simulink model "uas_sim"  (R2023a)
settings: Solver=VariableStepAuto  StartTime=0.0  StopTime=10.0  RelTol=1e-3  SampleTimeConstraint=STIndependent
values from neighbouring files (symbols this model uses):
  framePeriod_s = 1/frameRate_hz    (= 0.02)    [setup.m]
undefined symbols (not defined in the file or in its folder): Aircraft, datetime, datevec, Earth, Env, Fmu, InitCond, Telem, WGS84
libraries: aerolibconvert2 x8, simulink x8, aerolibadyn x3, aerolibasang x3, aerolibtransform2 x2, aerolibgravity2 x2, aerolibatmos2 x1, sharedutil x1, aerolibbdyn x1, shared6dof x1
(part 2 of 4)

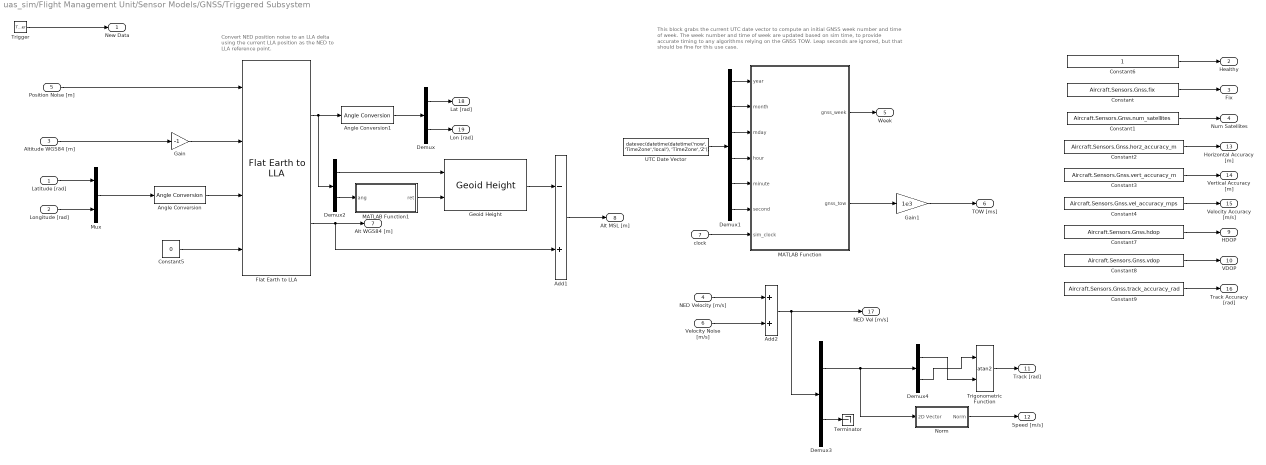
== system uas_sim/Flight Management Unit/Sensor Models/GNSS/Triggered Subsystem ==
  note: This block grabs the current UTC date vector to compute an initial GNSS week number
      | and time of week. The week number and time of week are updated based on sim time, to provide accurate timing to any algorithms relying on the GNSS TOW. Leap seconds are ignored, but that should be fine for this use case.
  note: Convert NED position noise to an LLA delta
      | using the current LLA position as the NED to
      | LLA reference point.
  Latitude [rad] : Inport
  "Longitude [rad] " : Inport  Port=2
  Altitude WGS84 [m] : Inport  Port=3
  NED Velocity [m/s] : Inport  Port=4  PortDimensions=3
  Position Noise [m] : Inport  Port=5  PortDimensions=3
  Velocity Noise [m/s] : Inport  Port=6  PortDimensions=3
  clock : Inport  Port=7
  Trigger : TriggerPort  VariantControl=Variant  ShowOutputPort=on
  Add1 : Sum  Inputs=-+
  Add2 : Sum
  Angle Conversion : aerolibconvert2/Angle Conversion  IU=rad  OU=deg
  Angle Conversion1 : aerolibconvert2/Angle Conversion  IU=deg  OU=rad
  Constant : Constant  Value=Aircraft.Sensors.Gnss.fix
  Constant1 : Constant  Value=Aircraft.Sensors.Gnss.num_satellites
  Constant2 : Constant  Value=Aircraft.Sensors.Gnss.horz_accuracy_m
  Constant3 : Constant  Value=Aircraft.Sensors.Gnss.vert_accuracy_m
  Constant4 : Constant  Value=Aircraft.Sensors.Gnss.vel_accuracy_mps
  Constant5 : Constant  Value=0
  Constant6 : Constant
  Constant7 : Constant  Value=Aircraft.Sensors.Gnss.hdop
  Constant8 : Constant  Value=Aircraft.Sensors.Gnss.vdop
  Constant9 : Constant  Value=Aircraft.Sensors.Gnss.track_accuracy_rad
  Demux : Demux  Outputs=2
  Demux1 : Demux  Outputs=6
  Demux2 : Demux  Outputs=2
  Demux3 : Demux  Outputs=[2 1]
  Demux4 : Demux  Outputs=2
  Flat Earth to LLA : aerolibtransform2/Flat Earth to LLA  units=Metric (MKS)  ptype=Earth (WGS84)  F=1/298.257223563  R=6378137  refPosPort=on  LL0=[0 10]  psi=0
  Gain : Gain  Gain=-1
  Gain1 : Gain  Gain=1e3
  Geoid Height : aerolibgravity2/Geoid Height  units=Metric (MKS)  gtype=EGM96  datafile='geoidegm96grid'  dtype=double  action=Warning
  MATLAB Function : MATLAB Function  TreatAsAtomicUnit=on
  MATLAB Function1 : MATLAB Function  TreatAsAtomicUnit=on
  Mux : Mux  Inputs=2
  Norm : Subsystem
  Terminator : Terminator
  Trigonometric Function : Trigonometry  Operator=atan2
  UTC Date Vector : Constant  Value=datevec(datetime(datetime('now', 'TimeZone','local'), 'TimeZone','Z'))  SampleTime=-1
  New Data : Outport
  Healthy : Outport  Port=2
  Fix : Outport  Port=3
  Num Satellites : Outport  Port=4
  Week : Outport  Port=5
  TOW [ms] : Outport  Port=6
  Alt WGS84 [m] : Outport  Port=7
  Alt MSL [m] : Outport  Port=8
  HDOP : Outport  Port=9
  VDOP : Outport  Port=10
  Track [rad] : Outport  Port=11
  Speed [m/s] : Outport  Port=12
  Horizontal Accuracy [m] : Outport  Port=13
  Vertical Accuracy [m] : Outport  Port=14
  Velocity Accuracy [m/s] : Outport  Port=15
  Track Accuracy [rad] : Outport  Port=16
  NED Vel [m/s] : Outport  Port=17
  Lat [rad] : Outport  Port=18
  Lon [rad] : Outport  Port=19
  wires:
  Constant/1 -> Fix/1
  Constant1/1 -> Num Satellites/1
  Constant2/1 -> Horizontal Accuracy [m]/1
  Constant3/1 -> Vertical Accuracy [m]/1
  Constant4/1 -> Velocity Accuracy [m/s]/1
  Position Noise [m]/1 -> Flat Earth to LLA/1
  Altitude WGS84 [m]/1 -> Gain/1
  Mux/1 -> Angle Conversion/1
  Angle Conversion/1 -> Flat Earth to LLA/3
  Constant5/1 -> Flat Earth to LLA/4
  "Longitude [rad] "/1 -> Mux/2
  Latitude [rad]/1 -> Mux/1
  Flat Earth to LLA/1 -> Demux2/1, Angle Conversion1/1
  Angle Conversion1/1 -> Demux/1
  Demux/2 -> Lon [rad]/1
  Demux/1 -> Lat [rad]/1
  Flat Earth to LLA/2 -> Add1/2, Alt WGS84 [m]/1
  NED Velocity [m/s]/1 -> Add2/1
  Add2/1 -> Demux3/1, NED Vel [m/s]/1
  Demux1/2 -> MATLAB Function/2(month)
  Demux1/6 -> MATLAB Function/6(second)
  UTC Date Vector/1 -> Demux1/1
  Demux1/1 -> MATLAB Function/1(year)
  Demux1/5 -> MATLAB Function/5(minute)
  Demux1/4 -> MATLAB Function/4(hour)
  Demux1/3 -> MATLAB Function/3(mday)
  MATLAB Function/2(gnss_tow) -> Gain1/1
  MATLAB Function/1(gnss_week) -> Week/1
  clock/1 -> MATLAB Function/7(sim_clock)
  Gain/1 -> Flat Earth to LLA/2
  Constant6/1 -> Healthy/1
  Trigger/1 -> New Data/1
  Gain1/1 -> TOW [ms]/1
  Demux2/1 -> Geoid Height/1
  Demux2/2 -> MATLAB Function1/1(ang)
  MATLAB Function1/1(ret) -> Geoid Height/2
  Geoid Height/1 -> Add1/1
  Add1/1 -> Alt MSL [m]/1
  Constant7/1 -> HDOP/1
  Constant8/1 -> VDOP/1
  Demux4/1 -> Trigonometric Function/2
  Demux4/2 -> Trigonometric Function/1
  Trigonometric Function/1 -> Track [rad]/1
  Velocity Noise [m/s]/1 -> Add2/2
  Constant9/1 -> Track Accuracy [rad]/1
  Demux3/1 -> Norm/1(2D Vector), Demux4/1
  Demux3/2 -> Terminator/1
  Norm/1(Norm) -> Speed [m/s]/1

== system uas_sim/Flight Management Unit/Sensor Models/IMU/Accelerometer ==
  Body Accel [m/s/s] : Inport  PortDimensions=3
  Gravitational Accel in Body Frame [m/s/s] : Inport  Port=2  PortDimensions=3
  Add : Sum  Inputs=+++
  Band-Limited White Noise : simulink/Sources/Band-Limited White Noise  Cov=Aircraft.Sensors.Imu.Accel.noise_mps2  Ts=0.1  seed=[23341]
  Constant : Constant  Value=Aircraft.Sensors.Imu.Accel.bias_mps2  VectorParams1D=off
  Constant1 : Constant  Value=Aircraft.Sensors.Imu.Accel.scale_factor
  Product : Product  Multiplication=Matrix(*)
  Reshape : Reshape  OutputDimensionality=Column vector (2-D)
  Reshape1 : Reshape  OutputDimensionality=Column vector (2-D)
  Reshape2 : Reshape
  Saturation : Saturate  UpperLimit=Aircraft.Sensors.Imu.Accel.upper_limit_mps2  LowerLimit=Aircraft.Sensors.Imu.Accel.lower_limit_mps2
  Subtract : Sum  Inputs=+-
  Accelerometer [m/s/s] : Outport  PortDimensions=3
  wires:
  Add/1 -> Saturation/1
  Band-Limited White Noise/1 -> Add/1
  Product/1 -> Add/3
  Constant/1 -> Add/2
  Constant1/1 -> Product/1
  Subtract/1 -> Product/2
  Reshape/1 -> Subtract/2
  Gravitational Accel in Body Frame [m/s/s]/1 -> Reshape/1
  Reshape1/1 -> Subtract/1
  Body Accel [m/s/s]/1 -> Reshape1/1
  Saturation/1 -> Reshape2/1
  Reshape2/1 -> Accelerometer [m/s/s]/1

== system uas_sim/Flight Management Unit/Sensor Models/IMU/Gyro ==
  Body Rotational Rate [rad/s] : Inport  PortDimensions=3
  Body Accel [m/s/s] : Inport  Port=2  PortDimensions=3
  Add1 : Sum  Inputs=++++
  Band-Limited White Noise : simulink/Sources/Band-Limited White Noise  Cov=Aircraft.Sensors.Imu.Gyro.noise_radps  Ts=0.1  seed=[23341]  VectorParams1D=off
  Constant1 : Constant  Value=Aircraft.Sensors.Imu.Gyro.bias_radps  VectorParams1D=off
  Constant2 : Constant  Value=Aircraft.Sensors.Imu.Gyro.accel_sens_radps
  Constant3 : Constant  Value=Aircraft.Sensors.Imu.Gyro.scale_factor  VectorParams1D=off
  Product : Product
  Product1 : Product  Multiplication=Matrix(*)
  Reshape : Reshape  OutputDimensionality=Column vector (2-D)
  Reshape1 : Reshape  OutputDimensionality=Column vector (2-D)
  Reshape2 : Reshape
  Saturation : Saturate  UpperLimit=Aircraft.Sensors.Imu.Gyro.upper_limit_radps  LowerLimit=Aircraft.Sensors.Imu.Gyro.lower_limit_radps
  Gyro [rad/s] : Outport  PortDimensions=3
  wires:
  Constant3/1 -> Product1/1
  Constant2/1 -> Product/1
  Add1/1 -> Saturation/1
  Constant1/1 -> Add1/3
  Product1/1 -> Add1/4
  Band-Limited White Noise/1 -> Add1/2
  Body Rotational Rate [rad/s]/1 -> Reshape/1
  Reshape/1 -> Product1/2
  Body Accel [m/s/s]/1 -> Product/2
  Product/1 -> Reshape1/1
  Reshape1/1 -> Add1/1
  Reshape2/1 -> Gyro [rad/s]/1
  Saturation/1 -> Reshape2/1

== system uas_sim/Flight Management Unit/Sensor Models/IMU/Magnetometer ==
  Body Magnetic Field [uT] : Inport  PortDimensions=3
  Add2 : Sum  Inputs=+++
  Band-Limited White Noise : simulink/Sources/Band-Limited White Noise  Cov=Aircraft.Sensors.Imu.Mag.noise_ut  Ts=0.1  seed=[23341]
  Constant1 : Constant  Value=Aircraft.Sensors.Imu.Mag.scale_factor  VectorParams1D=off
  Constant2 : Constant  Value=Aircraft.Sensors.Imu.Mag.bias_ut
  Product : Product  Multiplication=Matrix(*)
  Reshape : Reshape  OutputDimensionality=Column vector (2-D)
  Reshape1 : Reshape
  Saturation : Saturate  UpperLimit=Aircraft.Sensors.Imu.Mag.upper_limit_ut  LowerLimit=Aircraft.Sensors.Imu.Mag.lower_limit_ut
  Magnetometer [uT] : Outport  PortDimensions=3
  wires:
  Body Magnetic Field [uT]/1 -> Reshape/1
  Band-Limited White Noise/1 -> Add2/1
  Add2/1 -> Saturation/1
  Constant2/1 -> Add2/2
  Constant1/1 -> Product/1
  Reshape/1 -> Product/2
  Saturation/1 -> Reshape1/1
  Reshape1/1 -> Magnetometer [uT]/1
  Product/1 -> Add2/3

== system uas_sim/Flight Management Unit/Vehicle Management System (VMS)/Variant Subsystem/FMU v1 ==
  System Data : Inport
  Sensor Data : Inport  Port=2
  Navigation Filter Data : Inport  Port=3
  Telemetry Data : Inport  Port=4
  Flight Code : ModelReference  ModelNameDialog=fmu_v1.slx  SimulationMode=Normal  ModelReferenceVersion=2.2
  Virtual to Non-Virtual Mapping : Subsystem
  Virtual to Non-Virtual Mapping1 : Subsystem
  Virtual to Non-Virtual Mapping2 : Subsystem
  Virtual to Non-Virtual Mapping3 : Subsystem
  Virtual to Non-Virtual Mapping5 : Subsystem
  VMS Data : Outport
  wires:
  Telemetry Data/1 -> Virtual to Non-Virtual Mapping3/1(Virtual)
  Virtual to Non-Virtual Mapping2/1(Non-Virtual) -> Flight Code/3
  Virtual to Non-Virtual Mapping1/1(Non-Virtual) -> Flight Code/2
  Navigation Filter Data/1 -> Virtual to Non-Virtual Mapping2/1(Virtual)
  System Data/1 -> Virtual to Non-Virtual Mapping/1(Virtual)
  Flight Code/1 -> Virtual to Non-Virtual Mapping5/1(Non-Virtual)
  Virtual to Non-Virtual Mapping/1(Non-Virtual) -> Flight Code/1
  Virtual to Non-Virtual Mapping5/1(Virtual) -> VMS Data/1
  Sensor Data/1 -> Virtual to Non-Virtual Mapping1/1(Virtual)
  Virtual to Non-Virtual Mapping3/1(Non-Virtual) -> Flight Code/4

== system uas_sim/Flight Management Unit/Vehicle Management System (VMS)/Variant Subsystem/FMU v2 ==
  System Data : Inport
  Sensor Data : Inport  Port=2
  Navigation Filter Data : Inport  Port=3
  Telemetry Data : Inport  Port=4
  Flight Code : ModelReference  ModelNameDialog=fmu_v2.slx  SimulationMode=Normal  ModelReferenceVersion=4.2
  Virtual to Non-Virtual Mapping : Subsystem
  Virtual to Non-Virtual Mapping1 : Subsystem
  Virtual to Non-Virtual Mapping2 : Subsystem
  Virtual to Non-Virtual Mapping3 : Subsystem
  Virtual to Non-Virtual Mapping4 : Subsystem
  VMS Data : Outport
  wires:
  Virtual to Non-Virtual Mapping3/1(Non-Virtual) -> Flight Code/4
  Sensor Data/1 -> Virtual to Non-Virtual Mapping1/1(Virtual)
  Virtual to Non-Virtual Mapping4/1(Virtual) -> VMS Data/1
  Virtual to Non-Virtual Mapping/1(Non-Virtual) -> Flight Code/1
  Flight Code/1 -> Virtual to Non-Virtual Mapping4/1(Non-Virtual)
  System Data/1 -> Virtual to Non-Virtual Mapping/1(Virtual)
  Navigation Filter Data/1 -> Virtual to Non-Virtual Mapping2/1(Virtual)
  Virtual to Non-Virtual Mapping1/1(Non-Virtual) -> Flight Code/2
  Virtual to Non-Virtual Mapping2/1(Non-Virtual) -> Flight Code/3
  Telemetry Data/1 -> Virtual to Non-Virtual Mapping3/1(Virtual)

== system uas_sim/Flight Management Unit/Vehicle Management System (VMS)/Variant Subsystem/FMU v2 Beta ==
  System Data : Inport
  Sensor Data : Inport  Port=2
  Navigation Filter Data : Inport  Port=3
  Telemetry Data : Inport  Port=4
  Flight Code : ModelReference  ModelNameDialog=fmu_v2_beta.slx  SimulationMode=Normal  ModelReferenceVersion=2.5
  Virtual to Non-Virtual Mapping : Subsystem
  Virtual to Non-Virtual Mapping1 : Subsystem
  Virtual to Non-Virtual Mapping2 : Subsystem
  Virtual to Non-Virtual Mapping3 : Subsystem
  Virtual to Non-Virtual Mapping5 : Subsystem
  VMS Data : Outport
  wires:
  Virtual to Non-Virtual Mapping3/1(Non-Virtual) -> Flight Code/4
  Sensor Data/1 -> Virtual to Non-Virtual Mapping1/1(Virtual)
  Virtual to Non-Virtual Mapping5/1(Virtual) -> VMS Data/1
  Virtual to Non-Virtual Mapping/1(Non-Virtual) -> Flight Code/1
  Flight Code/1 -> Virtual to Non-Virtual Mapping5/1(Non-Virtual)
  System Data/1 -> Virtual to Non-Virtual Mapping/1(Virtual)
  Navigation Filter Data/1 -> Virtual to Non-Virtual Mapping2/1(Virtual)
  Virtual to Non-Virtual Mapping1/1(Non-Virtual) -> Flight Code/2
  Virtual to Non-Virtual Mapping2/1(Non-Virtual) -> Flight Code/3
  Telemetry Data/1 -> Virtual to Non-Virtual Mapping3/1(Virtual)

== system uas_sim/Vehicle/Forces and Moments/Aerodynamic/Aerodynamic Forces and Moments Coef Axis Variant ==
  Coef : Inport
  Dynamic Pressure [Pa] : Inport  Port=2
  Body Velocity [m/s] : Inport  Port=3
  Body Axis Coef : Subsystem  VariantControl=Aircraft.Aero.axis == 3
  Stability Axis Coef : Subsystem  VariantControl=Aircraft.Aero.axis == 2
  Wind Axis Coef : Subsystem  VariantControl=Aircraft.Aero.axis == 1
  Fxyz Mxyz : Outport

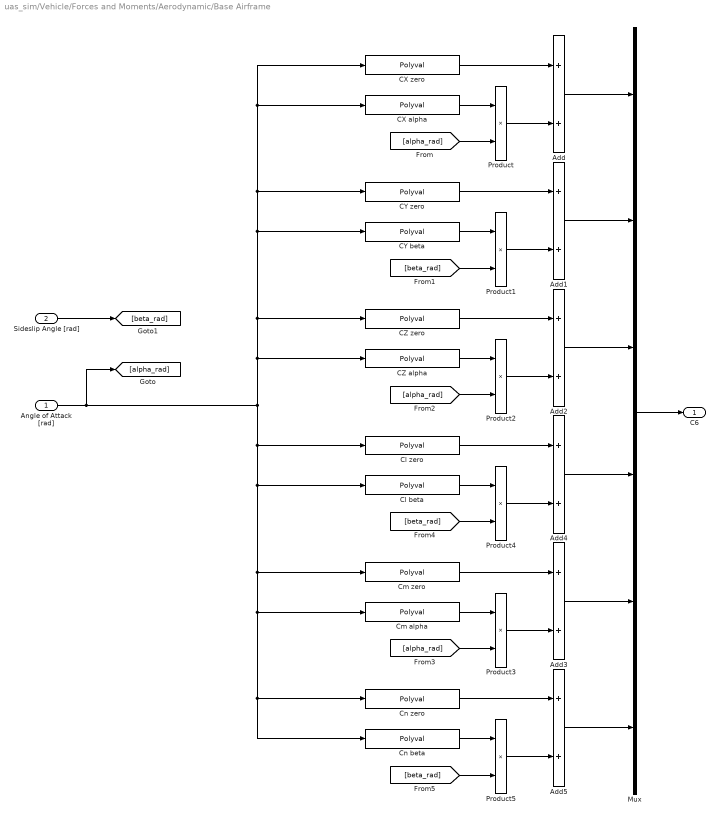
== system uas_sim/Vehicle/Forces and Moments/Aerodynamic/Base Airframe ==
  Angle of Attack [rad] : Inport
  Sideslip Angle [rad] : Inport  Port=2
  Add{,1..5} (6 alike) : Sum
  CX alpha : Polyval  Coefs=Aircraft.Aero.CX.alpha
  CX zero : Polyval  Coefs=Aircraft.Aero.CX.zero
  CY beta : Polyval  Coefs=Aircraft.Aero.CY.beta
  CY zero : Polyval  Coefs=Aircraft.Aero.CY.zero
  CZ alpha : Polyval  Coefs=Aircraft.Aero.CZ.alpha
  CZ zero : Polyval  Coefs=Aircraft.Aero.CZ.zero
  Cl beta : Polyval  Coefs=Aircraft.Aero.Cl.beta
  Cl zero : Polyval  Coefs=Aircraft.Aero.Cl.zero
  Cm alpha : Polyval  Coefs=Aircraft.Aero.Cm.alpha
  Cm zero : Polyval  Coefs=Aircraft.Aero.Cm.zero
  Cn beta : Polyval  Coefs=Aircraft.Aero.Cn.beta
  Cn zero : Polyval  Coefs=Aircraft.Aero.Cn.zero
  Mux : Mux  Inputs=6
  Product{,1..5} (6 alike) : Product
  C6 : Outport
  wires:
  Product/1 -> Add/2
  Add/1 -> Mux/1
  CX alpha/1 -> Product/1
  CX zero/1 -> Add/1
  Sideslip Angle [rad]/1 -> [beta_rad]
  [alpha_rad] -> Product/2
  Mux/1 -> C6/1
  [beta_rad] -> Product1/2
  CY zero/1 -> Add1/1
  CY beta/1 -> Product1/1
  Product1/1 -> Add1/2
  Add1/1 -> Mux/2
  CZ zero/1 -> Add2/1
  CZ alpha/1 -> Product2/1
  Add2/1 -> Mux/3
  Product2/1 -> Add2/2
  Product3/1 -> Add3/2
  Add3/1 -> Mux/5
  Cm alpha/1 -> Product3/1
  Cm zero/1 -> Add3/1
  [alpha_rad] -> Product2/2
  [alpha_rad] -> Product3/2
  Add4/1 -> Mux/4
  Product4/1 -> Add4/2
  Cl beta/1 -> Product4/1
  Cl zero/1 -> Add4/1
  [beta_rad] -> Product4/2
  [beta_rad] -> Product5/2
  Cn zero/1 -> Add5/1
  Cn beta/1 -> Product5/1
  Product5/1 -> Add5/2
  Add5/1 -> Mux/6
  Angle of Attack [rad]/1 -> [alpha_rad], Cl zero/1, Cl beta/1, Cm zero/1, Cm alpha/1, Cn zero/1, Cn beta/1, CZ alpha/1, CZ zero/1, CY beta/1, CY zero/1, CX alpha/1, CX zero/1

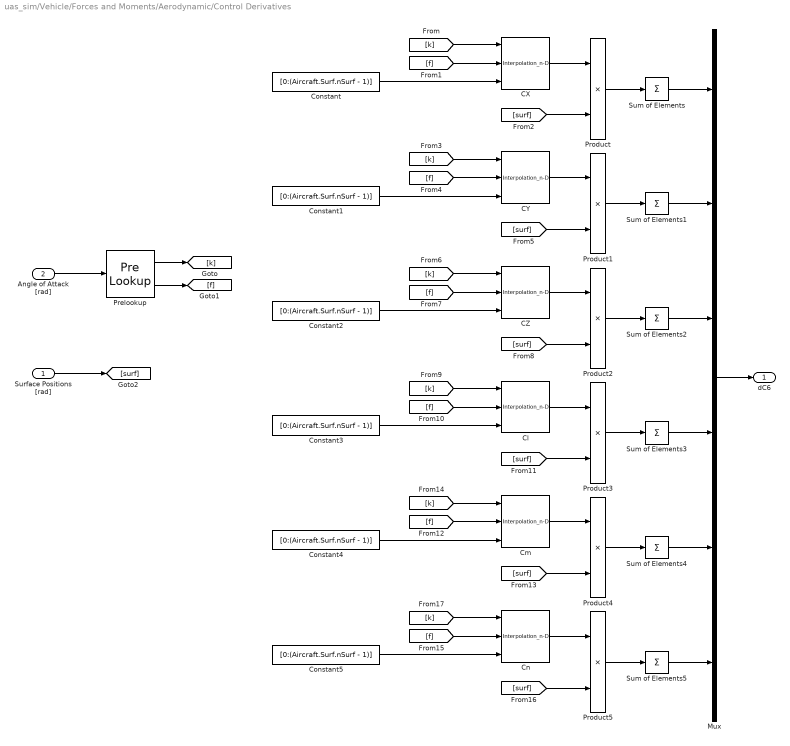
== system uas_sim/Vehicle/Forces and Moments/Aerodynamic/Control Derivatives ==
  Surface Positions [rad] : Inport
  Angle of Attack [rad] : Inport  Port=2
  CX : Interpolation_n-D  Table=Aircraft.Aero.CX.surf  DiagnosticForOutOfRangeInput=Warning  NumSelectionDims=1  InternalRulePriority=Speed
      settings: InputPortMap=u0,u1,u2
  CY : Interpolation_n-D  Table=Aircraft.Aero.CY.surf  DiagnosticForOutOfRangeInput=Warning  NumSelectionDims=1  InternalRulePriority=Speed
      settings: InputPortMap=u0,u1,u2
  CZ : Interpolation_n-D  Table=Aircraft.Aero.CZ.surf  DiagnosticForOutOfRangeInput=Warning  NumSelectionDims=1  InternalRulePriority=Speed
      settings: InputPortMap=u0,u1,u2
  Cl : Interpolation_n-D  Table=Aircraft.Aero.Cl.surf  DiagnosticForOutOfRangeInput=Warning  NumSelectionDims=1  InternalRulePriority=Speed
      settings: InputPortMap=u0,u1,u2
  Cm : Interpolation_n-D  Table=Aircraft.Aero.Cm.surf  DiagnosticForOutOfRangeInput=Warning  NumSelectionDims=1  InternalRulePriority=Speed
      settings: InputPortMap=u0,u1,u2
  Cn : Interpolation_n-D  Table=Aircraft.Aero.Cn.surf  DiagnosticForOutOfRangeInput=Warning  NumSelectionDims=1  InternalRulePriority=Speed
      settings: InputPortMap=u0,u1,u2
  Constant{,1..5} (6 alike) : Constant  Value=[0:(Aircraft.Surf.nSurf - 1)]
  Mux : Mux  Inputs=6
  Prelookup : PreLookup  BreakpointsData=Aircraft.Aero.CntrlEff.alpha  ExtrapMethod=Linear
  Product{,1..5} (6 alike) : Product
  Sum of Elements{,1..5} (6 alike) : Sum  Inputs=+
  dC6 : Outport
  wires:
  [k] -> Cm/1
  CY/1 -> Product1/1
  [f] -> Cn/2
  Product5/1 -> Sum of Elements5/1
  [surf] -> Product5/2
  Constant4/1 -> Cm/3
  Sum of Elements1/1 -> Mux/2
  [k] -> Cn/1
  Sum of Elements5/1 -> Mux/6
  Constant3/1 -> Cl/3
  [surf] -> Product3/2
  [k] -> Cl/1
  [f] -> Cl/2
  Constant2/1 -> CZ/3
  [k] -> CZ/1
  [surf] -> Product2/2
  Cl/1 -> Product3/1
  CZ/1 -> Product2/1
  Product2/1 -> Sum of Elements2/1
  Product3/1 -> Sum of Elements3/1
  Product1/1 -> Sum of Elements1/1
  Product/1 -> Sum of Elements/1
  [k] -> CY/1
  [f] -> CY/2
  Constant1/1 -> CY/3
  Constant/1 -> CX/3
  Cm/1 -> Product4/1
  [k] -> CX/1
  [surf] -> Product/2
  Prelookup/2 -> [f]
  Mux/1 -> dC6/1
  Prelookup/1 -> [k]
  Product4/1 -> Sum of Elements4/1
  Cn/1 -> Product5/1
  Angle of Attack [rad]/1 -> Prelookup/1
  Surface Positions [rad]/1 -> [surf]
  [f] -> CZ/2
  [f] -> Cm/2
  Sum of Elements2/1 -> Mux/3
  CX/1 -> Product/1
  [f] -> CX/2
  Constant5/1 -> Cn/3
  [surf] -> Product4/2
  Sum of Elements/1 -> Mux/1
  Sum of Elements4/1 -> Mux/5
  [surf] -> Product1/2
  Sum of Elements3/1 -> Mux/4

== system uas_sim/Vehicle/Forces and Moments/Aerodynamic/Dynamic Derivatives ==
  note: Divide by zero protection
  Airspeed [m/s] : Inport
  Body Rotational Rate [rad/s] : Inport  Port=2
  Angle of Attack [rad] : Inport  Port=3
  Add : Sum  Inputs=+++
  Constant : Constant  Value=Aircraft.Geom.b_m
  Constant1 : Constant  Value=Aircraft.Geom.c_m
  Constant2 : Constant  Value=Aircraft.Geom.b_m
  Demux : Demux  Outputs=3
  Divide : Product  Inputs=*/
  Gain : Gain  Gain=2
  Mux : Mux  Inputs=3
  Pitch Rate : Subsystem
  Product : Product
  Roll Rate : Subsystem
  Saturation : Saturate  UpperLimit=inf  LowerLimit=1e-3
  Yaw Rate : Subsystem
  dC6 : Outport
  wires:
  Constant/1 -> Mux/1
  Body Rotational Rate [rad/s]/1 -> Product/1
  Mux/1 -> Product/2
  Airspeed [m/s]/1 -> Gain/1
  Gain/1 -> Saturation/1
  Product/1 -> Divide/1
  Saturation/1 -> Divide/2
  Divide/1 -> Demux/1
  Demux/1 -> Roll Rate/2(p_hat)
  Demux/2 -> Pitch Rate/2(q_hat)
  Demux/3 -> Yaw Rate/2(r_hat)
  Angle of Attack [rad]/1 -> Yaw Rate/1(Angle of Attack [rad]), Pitch Rate/1(Angle of Attack [rad]), Roll Rate/1(Angle of Attack [rad])
  Roll Rate/1(dC6) -> Add/1
  Pitch Rate/1(dC6) -> Add/2
  Yaw Rate/1(dC6) -> Add/3
  Constant2/1 -> Mux/3
  Constant1/1 -> Mux/2
  Add/1 -> dC6/1

== system uas_sim/Vehicle/Forces and Moments/Propulsive/Motor ==
  note: RPM to rad/s
  Voltage [V] : Inport
  Motor Rotation Rate [rad/s] : Inport  Port=2
  Constant : Constant  Value=Aircraft.Motor.kv
  Constant1 : Constant  Value=Aircraft.Motor.io
  Divide : Product  Inputs=*/
  Divide2 : Product  Inputs=*/
  Gain : Gain  Gain=1/Aircraft.Motor.r
  Gain2 : Gain  Gain=2 * pi / 60
  Subtract : Sum  Inputs=+-
  Subtract1 : Sum  Inputs=+-
  Torque [N-m] : Outport
  wires:
  Gain2/1 -> [KvSI], Divide/2
  [KvSI] -> Divide2/2
  Constant1/1 -> Subtract1/2
  Motor Rotation Rate [rad/s]/1 -> Divide/1
  Divide/1 -> Subtract/2
  Constant/1 -> Gain2/1
  Gain/1 -> Subtract1/1
  Subtract1/1 -> Divide2/1
  Voltage [V]/1 -> Subtract/1
  Divide2/1 -> Torque [N-m]/1
  Subtract/1 -> Gain/1

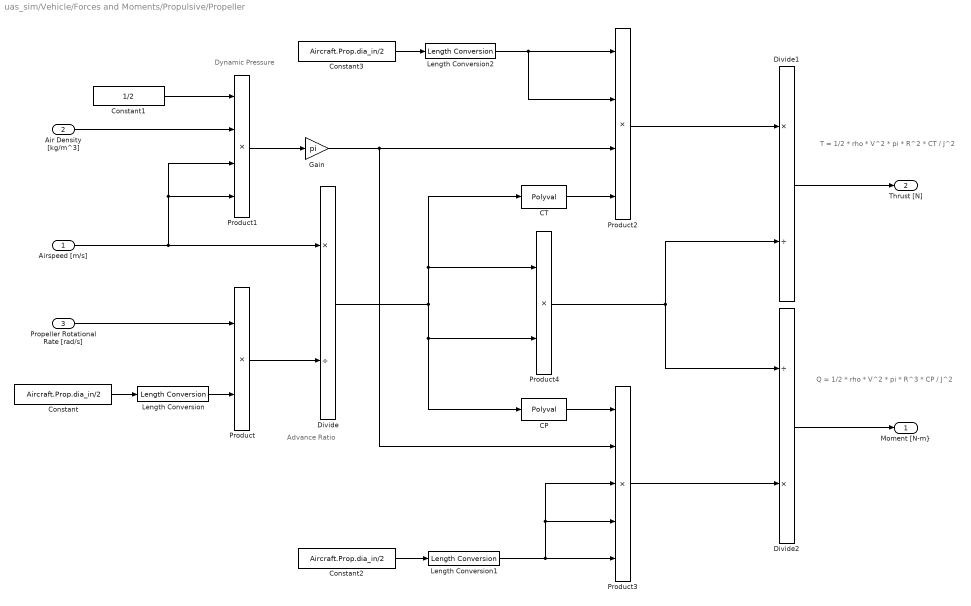
== system uas_sim/Vehicle/Forces and Moments/Propulsive/Propeller ==
  note: Dynamic Pressure
  note: Q = 1/2 * rho * V^2 * pi * R^3 * CP / J^2
  note: T = 1/2 * rho * V^2 * pi * R^2 * CT / J^2
  note: Advance Ratio
  Airspeed [m/s] : Inport
  Air Density [kg/m^3] : Inport  Port=2
  Propeller Rotational Rate [rad/s] : Inport  Port=3
  CP : Polyval  Coefs=Aircraft.prop.cp
  CT : Polyval  Coefs=Aircraft.prop.ct
  Constant : Constant  Value=Aircraft.Prop.dia_in/2
  Constant1 : Constant  Value=1/2
  Constant2 : Constant  Value=Aircraft.Prop.dia_in/2
  Constant3 : Constant  Value=Aircraft.Prop.dia_in/2
  Divide : Product  Inputs=*/
  Divide1 : Product  Inputs=*/
  Divide2 : Product  Inputs=/*
  Gain : Gain  Gain=pi
  Length Conversion : aerolibconvert2/Length Conversion  IU=in  OU=m
  Length Conversion1 : aerolibconvert2/Length Conversion  IU=in  OU=m
  Length Conversion2 : aerolibconvert2/Length Conversion  IU=in  OU=m
  Product : Product
  Product1 : Product  Inputs=4
  Product2 : Product  Inputs=4
  Product3 : Product  Inputs=5
  Product4 : Product
  "Moment [N-m}" : Outport
  Thrust [N] : Outport  Port=2
  wires:
  Divide2/1 -> "Moment [N-m}"/1
  Length Conversion/1 -> Product/2
  Product4/1 -> Divide2/1, Divide1/2
  Constant2/1 -> Length Conversion1/1
  Airspeed [m/s]/1 -> Divide/1, Product1/4, Product1/3
  Propeller Rotational Rate [rad/s]/1 -> Product/1
  Length Conversion1/1 -> Product3/4, Product3/3, Product3/5
  Product1/1 -> Gain/1
  Gain/1 -> Product3/2, Product2/3
  Air Density [kg/m^3]/1 -> Product1/2
  Divide1/1 -> Thrust [N]/1
  Product3/1 -> Divide2/2
  Constant1/1 -> Product1/1
  CP/1 -> Product3/1
  CT/1 -> Product2/4
  Product2/1 -> Divide1/1
  Length Conversion2/1 -> Product2/2, Product2/1
  Constant/1 -> Length Conversion/1
  Constant3/1 -> Length Conversion2/1
  Divide/1 -> Product4/2, CP/1, Product4/1, CT/1
  Product/1 -> Divide/2

== system uas_sim/Flight Management Unit/Sensor Models/GNSS/Triggered Subsystem/Norm ==
  2D Vector : Inport
  Product : Product
  Sqrt : Sqrt
  Sum of Elements : Sum  Inputs=+
  Norm : Outport
  wires:
  2D Vector/1 -> Product/2, Product/1
  Product/1 -> Sum of Elements/1
  Sum of Elements/1 -> Sqrt/1
  Sqrt/1 -> Norm/1

== system uas_sim/Flight Management Unit/Vehicle Management System (VMS)/Variant Subsystem/FMU v1/Virtual to Non-Virtual Mapping ==
  Virtual : Inport
  Bus Creator : BusCreator  Inputs=6  OutDataTypeStr=Bus: SysData  NonVirtualBus=on
  Bus Selector : BusSelector  OutputSignals=Frame Time [us],Input Voltage,Regulated Voltage,PWM Voltage,SBUS Voltage,System Time [us]
  Data Type Conversion : DataTypeConversion  OutDataTypeStr=int32  SaturateOnIntegerOverflow=off  RndMeth=Floor
  Data Type Conversion{1..4} (4 alike) : DataTypeConversion  OutDataTypeStr=single  SaturateOnIntegerOverflow=off  RndMeth=Floor
  Data Type Conversion5 : DataTypeConversion  OutDataTypeStr=int64  SaturateOnIntegerOverflow=off  RndMeth=Floor
  Non-Virtual : Outport  OutDataTypeStr=Bus: SysData
  wires:
  Data Type Conversion5/1 -> Bus Creator/6  "sys_time_us"
  Bus Selector/6 -> Data Type Conversion5/1  "<System Time [us]>"
  Data Type Conversion4/1 -> Bus Creator/5  "sbus_volt"
  Data Type Conversion3/1 -> Bus Creator/4  "pwm_volt"
  Data Type Conversion2/1 -> Bus Creator/3  "reg_volt"
  Bus Selector/5 -> Data Type Conversion4/1  "<SBUS Voltage>"
  Bus Selector/4 -> Data Type Conversion3/1  "<PWM Voltage>"
  Bus Selector/3 -> Data Type Conversion2/1  "<Regulated Voltage>"
  Data Type Conversion1/1 -> Bus Creator/2  "input_volt"
  Bus Selector/2 -> Data Type Conversion1/1  "<Input Voltage>"
  Data Type Conversion/1 -> Bus Creator/1  "frame_time_us"
  Bus Selector/1 -> Data Type Conversion/1  "<Frame Time [us]>"
  Virtual/1 -> Bus Selector/1
  Bus Creator/1 -> Non-Virtual/1

== system uas_sim/Flight Management Unit/Vehicle Management System (VMS)/Variant Subsystem/FMU v1/Virtual to Non-Virtual Mapping1 ==
  Virtual : Inport
  Bus Creator : BusCreator  Inputs=7  OutDataTypeStr=Bus: SensorData  NonVirtualBus=on
  Bus Selector : BusSelector  OutputSignals=Pitot Static Installed,Inceptor,IMU,GNSS,Static Pressure,Differential Pressure,Analog
  Data Type Conversion : DataTypeConversion  OutDataTypeStr=boolean  SaturateOnIntegerOverflow=off  RndMeth=Floor
  Virtual to Non-Virtual Mapping1 : Subsystem
  Virtual to Non-Virtual Mapping2 : Subsystem
  Virtual to Non-Virtual Mapping3 : Subsystem
  Virtual to Non-Virtual Mapping4 : Subsystem
  Virtual to Non-Virtual Mapping5 : Subsystem
  Virtual to Non-Virtual Mapping6 : Subsystem
  Non-Virtual : Outport  OutDataTypeStr=Bus: SensorData
  wires:
  Virtual/1 -> Bus Selector/1
  Bus Creator/1 -> Non-Virtual/1
  Bus Selector/1 -> Data Type Conversion/1  "<Pitot Static Installed>"
  Data Type Conversion/1 -> Bus Creator/1  "pitot_static_installed"
  Bus Selector/2 -> Virtual to Non-Virtual Mapping1/1(Virtual)  "<Inceptor>"
  Virtual to Non-Virtual Mapping1/1(Non-Virtual) -> Bus Creator/2  "inceptor"
  Virtual to Non-Virtual Mapping2/1(Non-Virtual) -> Bus Creator/3  "imu"
  Bus Selector/3 -> Virtual to Non-Virtual Mapping2/1(Virtual)  "<IMU>"
  Virtual to Non-Virtual Mapping3/1(Non-Virtual) -> Bus Creator/4  "gnss"
  Bus Selector/4 -> Virtual to Non-Virtual Mapping3/1(Virtual)  "<GNSS>"
  Virtual to Non-Virtual Mapping4/1(Non-Virtual) -> Bus Creator/5  "static_pres"
  Bus Selector/5 -> Virtual to Non-Virtual Mapping4/1(Virtual)  "<Static Pressure>"
  Virtual to Non-Virtual Mapping5/1(Non-Virtual) -> Bus Creator/6  "diff_pres"
  Bus Selector/6 -> Virtual to Non-Virtual Mapping5/1(Virtual)  "<Differential Pressure>"
  Bus Selector/7 -> Virtual to Non-Virtual Mapping6/1(Virtual)  "<Analog>"
  Virtual to Non-Virtual Mapping6/1(Non-Virtual) -> Bus Creator/7  "adc"

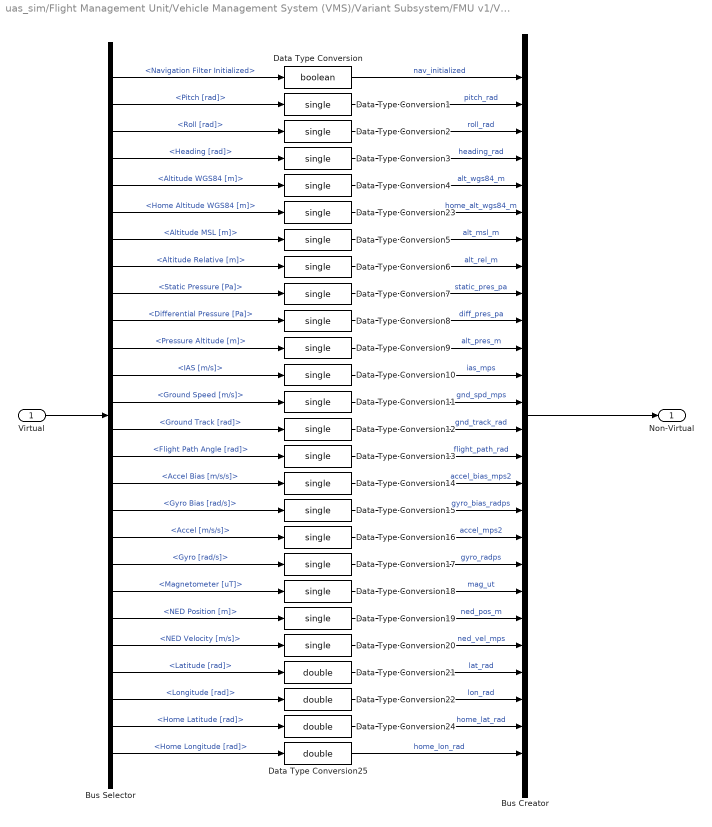
== system uas_sim/Flight Management Unit/Vehicle Management System (VMS)/Variant Subsystem/FMU v1/Virtual to Non-Virtual Mapping2 ==
  Virtual : Inport
  Bus Creator : BusCreator  Inputs=26  OutDataTypeStr=Bus: NavData  NonVirtualBus=on
  Bus Selector : BusSelector  OutputSignals=Navigation Filter Initialized,Pitch [rad],Roll [rad],Heading [rad],Altitude WGS84 [m],Home Altitude WGS84 [m],Altitude MSL [m],Altitude Relative [m],Static Pressure [Pa],Differential Pressure [Pa],Pressure Altitude [m],IAS [m/s],Ground Speed [m/s],Ground Track [rad],Flight Path Angle [rad],Accel Bias [m/s/s],Gyro Bias [rad/s],Accel [m/s/s],Gyro [rad/s],Magnetometer [uT],NED Position [m],NED Velocity [m/s],Latitude [rad],Longitude [rad],Home Latitude [rad],Home Longitude [rad]
  Data Type Conversion : DataTypeConversion  OutDataTypeStr=boolean  SaturateOnIntegerOverflow=off  RndMeth=Floor
  Data Type Conversion{1..20,23} (21 alike) : DataTypeConversion  OutDataTypeStr=single  SaturateOnIntegerOverflow=off  RndMeth=Floor
  Data Type Conversion{21..22,24..25} (4 alike) : DataTypeConversion  OutDataTypeStr=double  SaturateOnIntegerOverflow=off  RndMeth=Floor
  Non-Virtual : Outport  OutDataTypeStr=Bus: NavData
  wires:
  Virtual/1 -> Bus Selector/1
  Bus Creator/1 -> Non-Virtual/1
  Bus Selector/1 -> Data Type Conversion/1  "<Navigation Filter Initialized>"
  Bus Selector/2 -> Data Type Conversion1/1  "<Pitch [rad]>"
  Bus Selector/3 -> Data Type Conversion2/1  "<Roll [rad]>"
  Bus Selector/4 -> Data Type Conversion3/1  "<Heading [rad]>"
  Bus Selector/5 -> Data Type Conversion4/1  "<Altitude WGS84 [m]>"
  Bus Selector/7 -> Data Type Conversion5/1  "<Altitude MSL [m]>"
  Bus Selector/8 -> Data Type Conversion6/1  "<Altitude Relative [m]>"
  Bus Selector/9 -> Data Type Conversion7/1  "<Static Pressure [Pa]>"
  Bus Selector/10 -> Data Type Conversion8/1  "<Differential Pressure [Pa]>"
  Bus Selector/11 -> Data Type Conversion9/1  "<Pressure Altitude [m]>"
  Bus Selector/12 -> Data Type Conversion10/1  "<IAS [m/s]>"
  Bus Selector/13 -> Data Type Conversion11/1  "<Ground Speed [m/s]>"
  Bus Selector/14 -> Data Type Conversion12/1  "<Ground Track [rad]>"
  Bus Selector/15 -> Data Type Conversion13/1  "<Flight Path Angle [rad]>"
  Bus Selector/16 -> Data Type Conversion14/1  "<Accel Bias [m/s/s]>"
  Bus Selector/17 -> Data Type Conversion15/1  "<Gyro Bias [rad/s]>"
  Bus Selector/18 -> Data Type Conversion16/1  "<Accel [m/s/s]>"
  Bus Selector/19 -> Data Type Conversion17/1  "<Gyro [rad/s]>"
  Bus Selector/20 -> Data Type Conversion18/1  "<Magnetometer [uT]>"
  Bus Selector/21 -> Data Type Conversion19/1  "<NED Position [m]>"
  Bus Selector/22 -> Data Type Conversion20/1  "<NED Velocity [m/s]>"
  Bus Selector/23 -> Data Type Conversion21/1  "<Latitude [rad]>"
  Bus Selector/24 -> Data Type Conversion22/1  "<Longitude [rad]>"
  Data Type Conversion/1 -> Bus Creator/1  "nav_initialized"
  Data Type Conversion1/1 -> Bus Creator/2  "pitch_rad"
  Data Type Conversion2/1 -> Bus Creator/3  "roll_rad"
  Data Type Conversion3/1 -> Bus Creator/4  "heading_rad"
  Data Type Conversion4/1 -> Bus Creator/5  "alt_wgs84_m"
  Data Type Conversion22/1 -> Bus Creator/24  "lon_rad"
  Data Type Conversion21/1 -> Bus Creator/23  "lat_rad"
  Data Type Conversion20/1 -> Bus Creator/22  "ned_vel_mps"
  Data Type Conversion19/1 -> Bus Creator/21  "ned_pos_m"
  Data Type Conversion18/1 -> Bus Creator/20  "mag_ut"
  Data Type Conversion17/1 -> Bus Creator/19  "gyro_radps"
  Data Type Conversion16/1 -> Bus Creator/18  "accel_mps2"
  Data Type Conversion15/1 -> Bus Creator/17  "gyro_bias_radps"
  Data Type Conversion14/1 -> Bus Creator/16  "accel_bias_mps2"
  Data Type Conversion13/1 -> Bus Creator/15  "flight_path_rad"
  Data Type Conversion12/1 -> Bus Creator/14  "gnd_track_rad"
  Data Type Conversion11/1 -> Bus Creator/13  "gnd_spd_mps"
  Data Type Conversion10/1 -> Bus Creator/12  "ias_mps"
  Data Type Conversion9/1 -> Bus Creator/11  "alt_pres_m"
  Data Type Conversion8/1 -> Bus Creator/10  "diff_pres_pa"
  Data Type Conversion7/1 -> Bus Creator/9  "static_pres_pa"
  Data Type Conversion6/1 -> Bus Creator/8  "alt_rel_m"
  Data Type Conversion5/1 -> Bus Creator/7  "alt_msl_m"
  Bus Selector/6 -> Data Type Conversion23/1  "<Home Altitude WGS84 [m]>"
  Data Type Conversion23/1 -> Bus Creator/6  "home_alt_wgs84_m"
  Bus Selector/25 -> Data Type Conversion24/1  "<Home Latitude [rad]>"
  Bus Selector/26 -> Data Type Conversion25/1  "<Home Longitude [rad]>"
  Data Type Conversion24/1 -> Bus Creator/25  "home_lat_rad"
  Data Type Conversion25/1 -> Bus Creator/26  "home_lon_rad"

== system uas_sim/Flight Management Unit/Vehicle Management System (VMS)/Variant Subsystem/FMU v1/Virtual to Non-Virtual Mapping3 ==
  Virtual : Inport
  Bus Creator : BusCreator  Inputs=11  OutDataTypeStr=Bus: TelemData  NonVirtualBus=on
  Bus Selector : BusSelector  OutputSignals=Waypoints Updated,Fence Updated,Rally Points Updated,Current Waypoint Index,Number of Waypoints,Number of Fence Points,Number of Rally Points,Parameters,Flight Plan,Fence,Rally
  Data Type Conversion : DataTypeConversion  OutDataTypeStr=boolean  SaturateOnIntegerOverflow=off  RndMeth=Floor
  Data Type Conversion1 : DataTypeConversion  OutDataTypeStr=boolean  SaturateOnIntegerOverflow=off  RndMeth=Floor
  Data Type Conversion2 : DataTypeConversion  OutDataTypeStr=boolean  SaturateOnIntegerOverflow=off  RndMeth=Floor
  Data Type Conversion{3..6} (4 alike) : DataTypeConversion  OutDataTypeStr=int16  SaturateOnIntegerOverflow=off  RndMeth=Floor
  Data Type Conversion7 : DataTypeConversion  OutDataTypeStr=single  SaturateOnIntegerOverflow=off  RndMeth=Floor
  Signal Conversion : SignalConversion  ConversionOutput=Nonvirtual bus  OverrideOpt=off
  Signal Conversion1 : SignalConversion  ConversionOutput=Nonvirtual bus  OverrideOpt=off
  Signal Conversion2 : SignalConversion  ConversionOutput=Nonvirtual bus  OverrideOpt=off
  Non-Virtual : Outport  OutDataTypeStr=Bus: TelemData
  wires:
  Signal Conversion2/1 -> Bus Creator/11  "rally"
  Signal Conversion1/1 -> Bus Creator/10  "fence"
  Signal Conversion/1 -> Bus Creator/9  "flight_plan"
  Bus Selector/11 -> Signal Conversion2/1  "<Rally>"
  Bus Selector/10 -> Signal Conversion1/1  "<Fence>"
  Bus Selector/9 -> Signal Conversion/1  "<Flight Plan>"
  Data Type Conversion7/1 -> Bus Creator/8  "param"
  Data Type Conversion6/1 -> Bus Creator/7  "num_rally_points"
  Data Type Conversion5/1 -> Bus Creator/6  "num_fence_items"
  Data Type Conversion4/1 -> Bus Creator/5  "num_waypoints"
  Data Type Conversion3/1 -> Bus Creator/4  "current_waypoint"
  Data Type Conversion2/1 -> Bus Creator/3  "rally_points_updated"
  Data Type Conversion1/1 -> Bus Creator/2  "fence_updated"
  Data Type Conversion/1 -> Bus Creator/1  "waypoints_updated"
  Bus Selector/8 -> Data Type Conversion7/1  "<Parameters>"
  Bus Selector/7 -> Data Type Conversion6/1  "<Number of Rally Points>"
  Bus Selector/6 -> Data Type Conversion5/1  "<Number of Fence Points>"
  Bus Selector/5 -> Data Type Conversion4/1  "<Number of Waypoints>"
  Bus Selector/4 -> Data Type Conversion3/1  "<Current Waypoint Index>"
  Bus Selector/3 -> Data Type Conversion2/1  "<Rally Points Updated>"
  Bus Selector/2 -> Data Type Conversion1/1  "<Fence Updated>"
  Bus Selector/1 -> Data Type Conversion/1  "<Waypoints Updated>"
  Bus Creator/1 -> Non-Virtual/1
  Virtual/1 -> Bus Selector/1

== system uas_sim/Flight Management Unit/Vehicle Management System (VMS)/Variant Subsystem/FMU v1/Virtual to Non-Virtual Mapping5 ==
  Non-Virtual : Inport  OutDataTypeStr=Bus: VmsData
  Bus Creator : BusCreator  Inputs=8
  Bus Selector : BusSelector  OutputSignals=motors_enabled,waypoint_reached,mode,throttle_cmd_prcnt,aux,sbus,pwm,analog
  Data Type Conversion{,1..4} (5 alike) : DataTypeConversion  OutDataTypeStr=double  SaturateOnIntegerOverflow=off  RndMeth=Floor
  Subsystem2 : Subsystem
  Subsystem3 : Subsystem
  Subsystem4 : Subsystem
  Virtual : Outport
  wires:
  Non-Virtual/1 -> Bus Selector/1
  Bus Creator/1 -> Virtual/1
  Bus Selector/1 -> Data Type Conversion/1  "<motors_enabled>"
  Bus Selector/2 -> Data Type Conversion1/1  "<waypoint_reached>"
  Bus Selector/3 -> Data Type Conversion2/1  "<mode>"
  Bus Selector/4 -> Data Type Conversion3/1  "<throttle_cmd_prcnt>"
  Bus Selector/5 -> Data Type Conversion4/1  "<aux>"
  Data Type Conversion/1 -> Bus Creator/1  "Motors Enabled"
  Data Type Conversion1/1 -> Bus Creator/2  "Waypoint Reached"
  Data Type Conversion2/1 -> Bus Creator/3  "Mode"
  Data Type Conversion3/1 -> Bus Creator/4  "Throttle Cmd [%]"
  Data Type Conversion4/1 -> Bus Creator/5  "AUX"
  Bus Selector/6 -> Subsystem4/1(Non-Virtual)  "<sbus>"
  Bus Selector/7 -> Subsystem3/1(Non-Virtual)  "<pwm>"
  Bus Selector/8 -> Subsystem2/1(Non-Virtual)  "<analog>"
  Subsystem4/1(Virtual) -> Bus Creator/6  "SBUS"
  Subsystem3/1(Virtual) -> Bus Creator/7  "PWM"
  Subsystem2/1(Virtual) -> Bus Creator/8  "Analog"

== system uas_sim/Flight Management Unit/Vehicle Management System (VMS)/Variant Subsystem/FMU v2/Virtual to Non-Virtual Mapping ==
  Virtual : Inport
  Bus Creator : BusCreator  Inputs=2  OutDataTypeStr=Bus: SysData  NonVirtualBus=on
  Bus Selector : BusSelector  OutputSignals=Frame Time [us],System Time [us]
  Data Type Conversion : DataTypeConversion  OutDataTypeStr=int32  SaturateOnIntegerOverflow=off  RndMeth=Floor
  Data Type Conversion5 : DataTypeConversion  OutDataTypeStr=int64  SaturateOnIntegerOverflow=off  RndMeth=Floor
  Non-Virtual : Outport  OutDataTypeStr=Bus: SysData
  wires:
  Bus Creator/1 -> Non-Virtual/1
  Virtual/1 -> Bus Selector/1
  Bus Selector/1 -> Data Type Conversion/1  "<Frame Time [us]>"
  Data Type Conversion/1 -> Bus Creator/1  "frame_time_us"
  Bus Selector/2 -> Data Type Conversion5/1  "<System Time [us]>"
  Data Type Conversion5/1 -> Bus Creator/2  "sys_time_us"

== system uas_sim/Flight Management Unit/Vehicle Management System (VMS)/Variant Subsystem/FMU v2/Virtual to Non-Virtual Mapping1 ==
  Virtual : Inport
  Bus Creator : BusCreator  Inputs=8  OutDataTypeStr=Bus: SensorData  NonVirtualBus=on
  Bus Selector : BusSelector  OutputSignals=Pitot Static Installed,Inceptor,IMU,GNSS,Static Pressure,Differential Pressure,Analog,Battery
  Data Type Conversion : DataTypeConversion  OutDataTypeStr=boolean  SaturateOnIntegerOverflow=off  RndMeth=Floor
  Virtual to Non-Virtual Mapping1 : Subsystem
  Virtual to Non-Virtual Mapping2 : Subsystem
  Virtual to Non-Virtual Mapping3 : Subsystem
  Virtual to Non-Virtual Mapping4 : Subsystem
  Virtual to Non-Virtual Mapping5 : Subsystem
  Virtual to Non-Virtual Mapping6 : Subsystem
  Virtual to Non-Virtual Mapping7 : Subsystem
  Non-Virtual : Outport  OutDataTypeStr=Bus: SensorData
  wires:
  Virtual/1 -> Bus Selector/1
  Bus Creator/1 -> Non-Virtual/1
  Bus Selector/1 -> Data Type Conversion/1  "<Pitot Static Installed>"
  Data Type Conversion/1 -> Bus Creator/1  "pitot_static_installed"
  Bus Selector/2 -> Virtual to Non-Virtual Mapping1/1(Virtual)  "<Inceptor>"
  Virtual to Non-Virtual Mapping1/1(Non-Virtual) -> Bus Creator/2  "inceptor"
  Virtual to Non-Virtual Mapping2/1(Non-Virtual) -> Bus Creator/3  "imu"
  Bus Selector/3 -> Virtual to Non-Virtual Mapping2/1(Virtual)  "<IMU>"
  Virtual to Non-Virtual Mapping3/1(Non-Virtual) -> Bus Creator/4  "gnss"
  Bus Selector/4 -> Virtual to Non-Virtual Mapping3/1(Virtual)  "<GNSS>"
  Virtual to Non-Virtual Mapping4/1(Non-Virtual) -> Bus Creator/5  "static_pres"
  Bus Selector/5 -> Virtual to Non-Virtual Mapping4/1(Virtual)  "<Static Pressure>"
  Virtual to Non-Virtual Mapping5/1(Non-Virtual) -> Bus Creator/6  "diff_pres"
  Bus Selector/6 -> Virtual to Non-Virtual Mapping5/1(Virtual)  "<Differential Pressure>"
  Bus Selector/7 -> Virtual to Non-Virtual Mapping6/1(Virtual)  "<Analog>"
  Virtual to Non-Virtual Mapping6/1(Non-Virtual) -> Bus Creator/7  "adc"
  Virtual to Non-Virtual Mapping7/1(Non-Virtual) -> Bus Creator/8  "power_module"
  Bus Selector/8 -> Virtual to Non-Virtual Mapping7/1(Virtual)  "<Battery>"

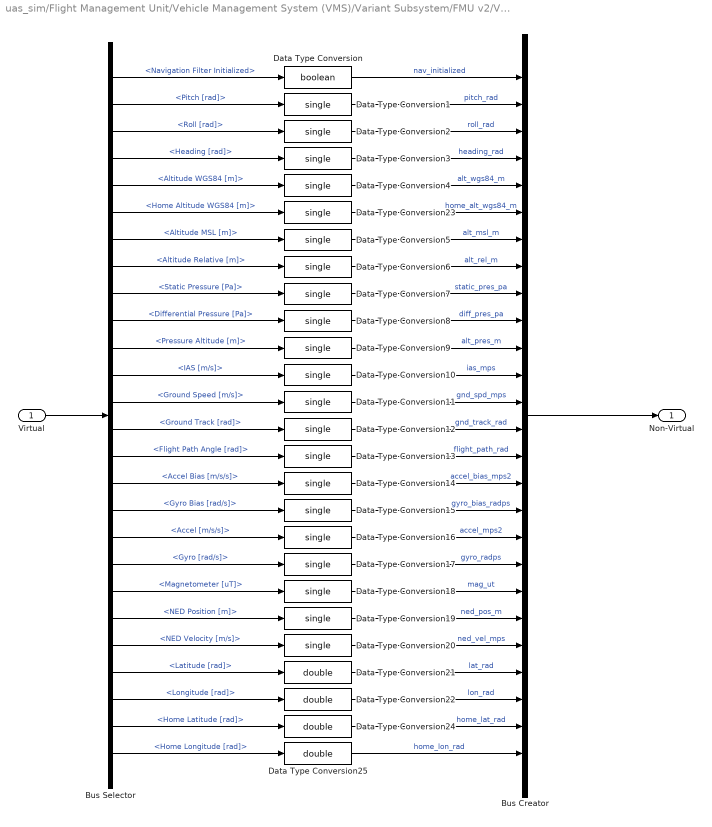
== system uas_sim/Flight Management Unit/Vehicle Management System (VMS)/Variant Subsystem/FMU v2/Virtual to Non-Virtual Mapping2 ==
  Virtual : Inport
  Bus Creator : BusCreator  Inputs=26  OutDataTypeStr=Bus: NavData  NonVirtualBus=on
  Bus Selector : BusSelector  OutputSignals=Navigation Filter Initialized,Pitch [rad],Roll [rad],Heading [rad],Altitude WGS84 [m],Home Altitude WGS84 [m],Altitude MSL [m],Altitude Relative [m],Static Pressure [Pa],Differential Pressure [Pa],Pressure Altitude [m],IAS [m/s],Ground Speed [m/s],Ground Track [rad],Flight Path Angle [rad],Accel Bias [m/s/s],Gyro Bias [rad/s],Accel [m/s/s],Gyro [rad/s],Magnetometer [uT],NED Position [m],NED Velocity [m/s],Latitude [rad],Longitude [rad],Home Latitude [rad],Home Longitude [rad]
  Data Type Conversion : DataTypeConversion  OutDataTypeStr=boolean  SaturateOnIntegerOverflow=off  RndMeth=Floor
  Data Type Conversion{1..20,23} (21 alike) : DataTypeConversion  OutDataTypeStr=single  SaturateOnIntegerOverflow=off  RndMeth=Floor
  Data Type Conversion{21..22,24..25} (4 alike) : DataTypeConversion  OutDataTypeStr=double  SaturateOnIntegerOverflow=off  RndMeth=Floor
  Non-Virtual : Outport  OutDataTypeStr=Bus: NavData
  wires:
  Virtual/1 -> Bus Selector/1
  Bus Creator/1 -> Non-Virtual/1
  Bus Selector/1 -> Data Type Conversion/1  "<Navigation Filter Initialized>"
  Bus Selector/2 -> Data Type Conversion1/1  "<Pitch [rad]>"
  Bus Selector/3 -> Data Type Conversion2/1  "<Roll [rad]>"
  Bus Selector/4 -> Data Type Conversion3/1  "<Heading [rad]>"
  Bus Selector/5 -> Data Type Conversion4/1  "<Altitude WGS84 [m]>"
  Bus Selector/7 -> Data Type Conversion5/1  "<Altitude MSL [m]>"
  Bus Selector/8 -> Data Type Conversion6/1  "<Altitude Relative [m]>"
  Bus Selector/9 -> Data Type Conversion7/1  "<Static Pressure [Pa]>"
  Bus Selector/10 -> Data Type Conversion8/1  "<Differential Pressure [Pa]>"
  Bus Selector/11 -> Data Type Conversion9/1  "<Pressure Altitude [m]>"
  Bus Selector/12 -> Data Type Conversion10/1  "<IAS [m/s]>"
  Bus Selector/13 -> Data Type Conversion11/1  "<Ground Speed [m/s]>"
  Bus Selector/14 -> Data Type Conversion12/1  "<Ground Track [rad]>"
  Bus Selector/15 -> Data Type Conversion13/1  "<Flight Path Angle [rad]>"
  Bus Selector/16 -> Data Type Conversion14/1  "<Accel Bias [m/s/s]>"
  Bus Selector/17 -> Data Type Conversion15/1  "<Gyro Bias [rad/s]>"
  Bus Selector/18 -> Data Type Conversion16/1  "<Accel [m/s/s]>"
  Bus Selector/19 -> Data Type Conversion17/1  "<Gyro [rad/s]>"
  Bus Selector/20 -> Data Type Conversion18/1  "<Magnetometer [uT]>"
  Bus Selector/21 -> Data Type Conversion19/1  "<NED Position [m]>"
  Bus Selector/22 -> Data Type Conversion20/1  "<NED Velocity [m/s]>"
  Bus Selector/23 -> Data Type Conversion21/1  "<Latitude [rad]>"
  Bus Selector/24 -> Data Type Conversion22/1  "<Longitude [rad]>"
  Data Type Conversion/1 -> Bus Creator/1  "nav_initialized"
  Data Type Conversion1/1 -> Bus Creator/2  "pitch_rad"
  Data Type Conversion2/1 -> Bus Creator/3  "roll_rad"
  Data Type Conversion3/1 -> Bus Creator/4  "heading_rad"
  Data Type Conversion4/1 -> Bus Creator/5  "alt_wgs84_m"
  Data Type Conversion22/1 -> Bus Creator/24  "lon_rad"
  Data Type Conversion21/1 -> Bus Creator/23  "lat_rad"
  Data Type Conversion20/1 -> Bus Creator/22  "ned_vel_mps"
  Data Type Conversion19/1 -> Bus Creator/21  "ned_pos_m"
  Data Type Conversion18/1 -> Bus Creator/20  "mag_ut"
  Data Type Conversion17/1 -> Bus Creator/19  "gyro_radps"
  Data Type Conversion16/1 -> Bus Creator/18  "accel_mps2"
  Data Type Conversion15/1 -> Bus Creator/17  "gyro_bias_radps"
  Data Type Conversion14/1 -> Bus Creator/16  "accel_bias_mps2"
  Data Type Conversion13/1 -> Bus Creator/15  "flight_path_rad"
  Data Type Conversion12/1 -> Bus Creator/14  "gnd_track_rad"
  Data Type Conversion11/1 -> Bus Creator/13  "gnd_spd_mps"
  Data Type Conversion10/1 -> Bus Creator/12  "ias_mps"
  Data Type Conversion9/1 -> Bus Creator/11  "alt_pres_m"
  Data Type Conversion8/1 -> Bus Creator/10  "diff_pres_pa"
  Data Type Conversion7/1 -> Bus Creator/9  "static_pres_pa"
  Data Type Conversion6/1 -> Bus Creator/8  "alt_rel_m"
  Data Type Conversion5/1 -> Bus Creator/7  "alt_msl_m"
  Bus Selector/6 -> Data Type Conversion23/1  "<Home Altitude WGS84 [m]>"
  Data Type Conversion23/1 -> Bus Creator/6  "home_alt_wgs84_m"
  Bus Selector/25 -> Data Type Conversion24/1  "<Home Latitude [rad]>"
  Bus Selector/26 -> Data Type Conversion25/1  "<Home Longitude [rad]>"
  Data Type Conversion24/1 -> Bus Creator/25  "home_lat_rad"
  Data Type Conversion25/1 -> Bus Creator/26  "home_lon_rad"

== system uas_sim/Flight Management Unit/Vehicle Management System (VMS)/Variant Subsystem/FMU v2/Virtual to Non-Virtual Mapping3 ==
  Virtual : Inport
  Bus Creator : BusCreator  Inputs=11  OutDataTypeStr=Bus: TelemData  NonVirtualBus=on
  Bus Selector : BusSelector  OutputSignals=Waypoints Updated,Fence Updated,Rally Points Updated,Current Waypoint Index,Number of Waypoints,Number of Fence Points,Number of Rally Points,Parameters,Flight Plan,Fence,Rally
  Data Type Conversion : DataTypeConversion  OutDataTypeStr=boolean  SaturateOnIntegerOverflow=off  RndMeth=Floor
  Data Type Conversion1 : DataTypeConversion  OutDataTypeStr=boolean  SaturateOnIntegerOverflow=off  RndMeth=Floor
  Data Type Conversion2 : DataTypeConversion  OutDataTypeStr=boolean  SaturateOnIntegerOverflow=off  RndMeth=Floor
  Data Type Conversion{3..6} (4 alike) : DataTypeConversion  OutDataTypeStr=int16  SaturateOnIntegerOverflow=off  RndMeth=Floor
  Data Type Conversion7 : DataTypeConversion  OutDataTypeStr=single  SaturateOnIntegerOverflow=off  RndMeth=Floor
  Signal Conversion : SignalConversion  ConversionOutput=Nonvirtual bus  OverrideOpt=off
  Signal Conversion1 : SignalConversion  ConversionOutput=Nonvirtual bus  OverrideOpt=off
  Signal Conversion2 : SignalConversion  ConversionOutput=Nonvirtual bus  OverrideOpt=off
  Non-Virtual : Outport  OutDataTypeStr=Bus: TelemData
  wires:
  Virtual/1 -> Bus Selector/1
  Bus Creator/1 -> Non-Virtual/1
  Bus Selector/1 -> Data Type Conversion/1  "<Waypoints Updated>"
  Bus Selector/2 -> Data Type Conversion1/1  "<Fence Updated>"
  Bus Selector/3 -> Data Type Conversion2/1  "<Rally Points Updated>"
  Bus Selector/4 -> Data Type Conversion3/1  "<Current Waypoint Index>"
  Bus Selector/5 -> Data Type Conversion4/1  "<Number of Waypoints>"
  Bus Selector/6 -> Data Type Conversion5/1  "<Number of Fence Points>"
  Bus Selector/7 -> Data Type Conversion6/1  "<Number of Rally Points>"
  Bus Selector/8 -> Data Type Conversion7/1  "<Parameters>"
  Data Type Conversion/1 -> Bus Creator/1  "waypoints_updated"
  Data Type Conversion1/1 -> Bus Creator/2  "fence_updated"
  Data Type Conversion2/1 -> Bus Creator/3  "rally_points_updated"
  Data Type Conversion3/1 -> Bus Creator/4  "current_waypoint"
  Data Type Conversion4/1 -> Bus Creator/5  "num_waypoints"
  Data Type Conversion5/1 -> Bus Creator/6  "num_fence_items"
  Data Type Conversion6/1 -> Bus Creator/7  "num_rally_points"
  Data Type Conversion7/1 -> Bus Creator/8  "param"
  Bus Selector/9 -> Signal Conversion/1  "<Flight Plan>"
  Bus Selector/10 -> Signal Conversion1/1  "<Fence>"
  Bus Selector/11 -> Signal Conversion2/1  "<Rally>"
  Signal Conversion/1 -> Bus Creator/9  "flight_plan"
  Signal Conversion1/1 -> Bus Creator/10  "fence"
  Signal Conversion2/1 -> Bus Creator/11  "rally"

== system uas_sim/Flight Management Unit/Vehicle Management System (VMS)/Variant Subsystem/FMU v2/Virtual to Non-Virtual Mapping4 ==
  Non-Virtual : Inport  OutDataTypeStr=Bus: VmsData
  Bus Creator : BusCreator  Inputs=9
  Bus Selector : BusSelector  OutputSignals=motors_enabled,waypoint_reached,mode,throttle_cmd_prcnt,aux,sbus,pwm,analog,battery
  Data Type Conversion{,1..4} (5 alike) : DataTypeConversion  OutDataTypeStr=double  SaturateOnIntegerOverflow=off  RndMeth=Floor
  Subsystem1 : Subsystem
  Subsystem2 : Subsystem
  Subsystem3 : Subsystem
  Subsystem4 : Subsystem
  Virtual : Outport
  wires:
  Non-Virtual/1 -> Bus Selector/1
  Bus Creator/1 -> Virtual/1
  Bus Selector/1 -> Data Type Conversion/1  "<motors_enabled>"
  Bus Selector/2 -> Data Type Conversion1/1  "<waypoint_reached>"
  Bus Selector/3 -> Data Type Conversion2/1  "<mode>"
  Bus Selector/4 -> Data Type Conversion3/1  "<throttle_cmd_prcnt>"
  Bus Selector/5 -> Data Type Conversion4/1  "<aux>"
  Data Type Conversion/1 -> Bus Creator/1  "Motors Enabled"
  Data Type Conversion1/1 -> Bus Creator/2  "Waypoint Reached"
  Data Type Conversion2/1 -> Bus Creator/3  "Mode"
  Data Type Conversion3/1 -> Bus Creator/4  "Throttle Cmd [%]"
  Data Type Conversion4/1 -> Bus Creator/5  "AUX"
  Bus Selector/6 -> Subsystem4/1(Non-Virtual)  "<sbus>"
  Bus Selector/7 -> Subsystem3/1(Non-Virtual)  "<pwm>"
  Bus Selector/8 -> Subsystem2/1(Non-Virtual)  "<analog>"
  Bus Selector/9 -> Subsystem1/1(Non-Virtual)  "<battery>"
  Subsystem4/1(Virtual) -> Bus Creator/6  "SBUS"
  Subsystem3/1(Virtual) -> Bus Creator/7  "PWM"
  Subsystem2/1(Virtual) -> Bus Creator/8  "Analog"
  Subsystem1/1(Virtual) -> Bus Creator/9  "Battery"

== system uas_sim/Flight Management Unit/Vehicle Management System (VMS)/Variant Subsystem/FMU v2 Beta/Virtual to Non-Virtual Mapping ==
  Virtual : Inport
  Bus Creator : BusCreator  Inputs=2  OutDataTypeStr=Bus: SysData  NonVirtualBus=on
  Bus Selector : BusSelector  OutputSignals=Frame Time [us],System Time [us]
  Data Type Conversion : DataTypeConversion  OutDataTypeStr=int32  SaturateOnIntegerOverflow=off  RndMeth=Floor
  Data Type Conversion5 : DataTypeConversion  OutDataTypeStr=int64  SaturateOnIntegerOverflow=off  RndMeth=Floor
  Non-Virtual : Outport  OutDataTypeStr=Bus: SysData
  wires:
  Bus Creator/1 -> Non-Virtual/1
  Virtual/1 -> Bus Selector/1
  Bus Selector/1 -> Data Type Conversion/1  "<Frame Time [us]>"
  Data Type Conversion/1 -> Bus Creator/1  "frame_time_us"
  Bus Selector/2 -> Data Type Conversion5/1  "<System Time [us]>"
  Data Type Conversion5/1 -> Bus Creator/2  "sys_time_us"

== system uas_sim/Flight Management Unit/Vehicle Management System (VMS)/Variant Subsystem/FMU v2 Beta/Virtual to Non-Virtual Mapping1 ==
  Virtual : Inport
  Bus Creator : BusCreator  Inputs=7  OutDataTypeStr=Bus: SensorData  NonVirtualBus=on
  Bus Selector : BusSelector  OutputSignals=Pitot Static Installed,Inceptor,IMU,GNSS,Static Pressure,Differential Pressure,Analog
  Data Type Conversion : DataTypeConversion  OutDataTypeStr=boolean  SaturateOnIntegerOverflow=off  RndMeth=Floor
  Virtual to Non-Virtual Mapping1 : Subsystem
  Virtual to Non-Virtual Mapping2 : Subsystem
  Virtual to Non-Virtual Mapping3 : Subsystem
  Virtual to Non-Virtual Mapping4 : Subsystem
  Virtual to Non-Virtual Mapping5 : Subsystem
  Virtual to Non-Virtual Mapping6 : Subsystem
  Non-Virtual : Outport  OutDataTypeStr=Bus: SensorData
  wires:
  Virtual/1 -> Bus Selector/1
  Bus Creator/1 -> Non-Virtual/1
  Bus Selector/1 -> Data Type Conversion/1  "<Pitot Static Installed>"
  Data Type Conversion/1 -> Bus Creator/1  "pitot_static_installed"
  Bus Selector/2 -> Virtual to Non-Virtual Mapping1/1(Virtual)  "<Inceptor>"
  Virtual to Non-Virtual Mapping1/1(Non-Virtual) -> Bus Creator/2  "inceptor"
  Virtual to Non-Virtual Mapping2/1(Non-Virtual) -> Bus Creator/3  "imu"
  Bus Selector/3 -> Virtual to Non-Virtual Mapping2/1(Virtual)  "<IMU>"
  Virtual to Non-Virtual Mapping3/1(Non-Virtual) -> Bus Creator/4  "gnss"
  Bus Selector/4 -> Virtual to Non-Virtual Mapping3/1(Virtual)  "<GNSS>"
  Virtual to Non-Virtual Mapping4/1(Non-Virtual) -> Bus Creator/5  "static_pres"
  Bus Selector/5 -> Virtual to Non-Virtual Mapping4/1(Virtual)  "<Static Pressure>"
  Virtual to Non-Virtual Mapping5/1(Non-Virtual) -> Bus Creator/6  "diff_pres"
  Bus Selector/6 -> Virtual to Non-Virtual Mapping5/1(Virtual)  "<Differential Pressure>"
  Bus Selector/7 -> Virtual to Non-Virtual Mapping6/1(Virtual)  "<Analog>"
  Virtual to Non-Virtual Mapping6/1(Non-Virtual) -> Bus Creator/7  "adc"
